simulink model "yori_tugas_variabel_m"  (R2023a)
settings: Solver=VariableStepAuto  StartTime=0.0  StopTime=100  RelTol=1e-3
values from neighbouring files (symbols this model uses):
  c = 6    [tugas_matlab_yori.mat]
  dxdt_init = 0    [tugas_matlab_yori.mat]
  k = 4    [tugas_matlab_yori.mat]
  m = 25    [tugas_matlab_yori.mat]
  t_step_F = 75    [tugas_matlab_yori.mat]
  t_stop = 100    [tugas_matlab_yori.mat]
  x_init = 5    [tugas_matlab_yori.mat]
settings Model: Creator=HP  LastModifiedBy=HP

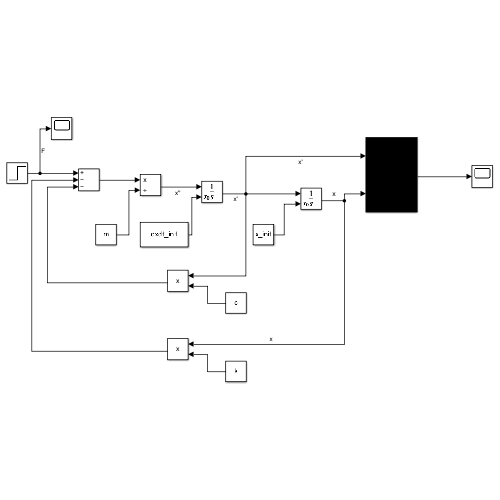
[thumbnail: Simulink's stored preview of the top-level diagram]
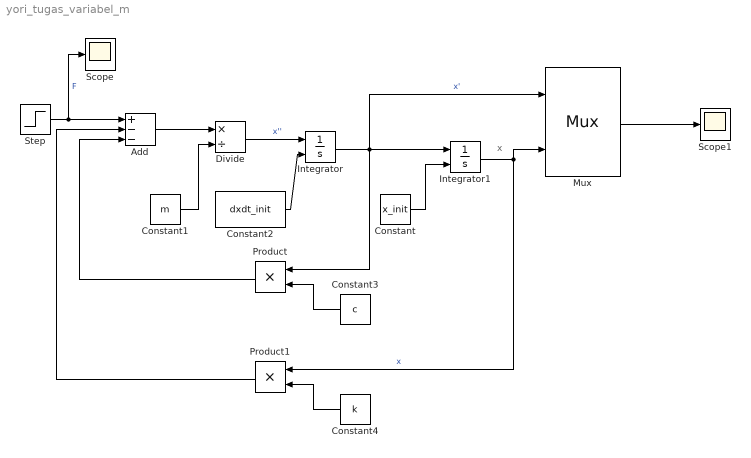
== system yori_tugas_variabel_m ==
  note: x
  Add : Sum  Inputs=+--
  Constant : Constant  Value=x_init
  Constant1 : Constant  Value=m
  Constant2 : Constant  Value=dxdt_init
  Constant3 : Constant  Value=c
  Constant4 : Constant  Value=k
  Divide : Product  Inputs=*/
  Integrator : Integrator  InitialConditionSource=external
  Integrator1 : Integrator  InitialConditionSource=external
  Mux : Mux  Inputs=2
  Product : Product
  Product1 : Product
  Scope : Scope
  Scope1 : Scope
  Step : Step  Time=t_step_F  After=t_stop  SampleTime=0
  wires:
  Constant2/1 -> Integrator/2
  Product1/1 -> Add/2
  Constant4/1 -> Product1/2
  Constant3/1 -> Product/2
  Constant/1 -> Integrator1/2
  Mux/1 -> Scope1/1
  Integrator/1 -> Product/1, Integrator1/1, Mux/1  "x'"
  Product/1 -> Add/3
  Step/1 -> Add/1, Scope/1  "F"
  Add/1 -> Divide/1
  Constant1/1 -> Divide/2
  Divide/1 -> Integrator/1  "x''"
  Integrator1/1 -> Mux/2, Product1/1  "x"
